simulink model "VehicleTest"  (Simulink 4.00)
settings: Solver=FixedStepDiscrete  StartTime=0.0  StopTime=GlobalStopTime  FixedStep=GlobalSampleTime  RelTol=1e-3
undefined symbols (not defined in the file): EntityTypes, g_EnableTarget, g_VehicleInputFiles, GlobalSampleTime, GSensorRollLimitDeg, OptionSaveDataAVDS, OptionSaveDataPlot, TargetStates, WaypointDefinitions
settings Model: Creator=mitchejw  LastModifiedBy=rasmussj  SaveTime=off  SaveOutput=off  ExtModeAutoUpdateStatusClock=off

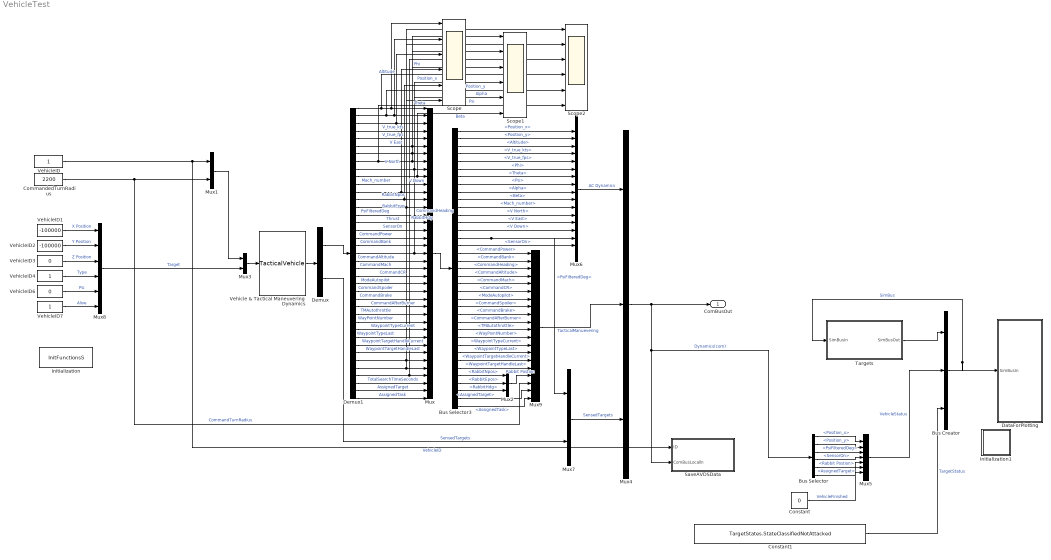
== system VehicleTest ==
  Bus Creator : BusCreator  Inputs=3
  Bus Selector : BusSelector  OutputSignals=AC Dynamics.Position_x,AC Dynamics.Position_y,AC Dynamics.PsiFilteredDeg,AC Dynamics.SensorOn,TacticalManuevering.Rabbit Postion,TacticalManuevering.AssignedTarget  MuxedOutput=off
  Bus Selector3 : BusSelector  OutputSignals=Position_x,Position_y,Altitude,V_true_kts,V_true_fps,Phi,Theta,Psi,Alpha,Beta,Mach_number,V North,V East,V Down,PsiFilteredDeg,SensorOn,CommandPower,CommandBank,CommandHeading,CommandAltitude,CommandMach,CommandCR,ModeAutopilot,CommandSpoiler,CommandBrake,CommandAfterBurner,TMAutothrottle,WayPointNumber,WaypointTypeCurrent,WaypointTypeLast,WaypointTargetHandleCurrent,WaypointTargetHandleLast,RabbitNpos,RabbitEpos,RabbitHdg,AssignedTarget,AssignedTask  MuxedOutput=off
  CommandedTurnRadius : Constant  Value=2200
  Constant : Constant  Value=0
  Constant1 : Constant  Value=TargetStates.StateClassifiedNotAttacked
  DataForPlotting : Subsystem  Priority=5
      settings: RTWFcnNameOpts=Auto  RTWFileNameOpts=Auto
  Demux : Demux  Outputs=[39 1]  BusSelectionMode=off
  Demux1 : Demux  Outputs=39  BusSelectionMode=off
  Initialization : S-Function  FunctionName=InitFunctionsS  PortCounts=[]  SFunctionModules=''
  Initialization1 : Subsystem  Priority=1
      settings: RTWFcnNameOpts=Auto  RTWFileNameOpts=Auto
  Mux : Mux  Inputs="[1 1 1 1 1 1 1 1 1 1 1 1 1 1 1 1 1 1 1 1  1 1 1 1 1 1 1 1 1 1  1 1 1 1 1 1 1 1 1]"
  Mux1 : Mux  Inputs=2
  Mux2 : Mux  Inputs=3
  Mux3 : Mux  Inputs=2
  Mux4 : Mux  Inputs=3
  Mux5 : Mux  Inputs=7
  Mux6 : Mux  Inputs=16
  Mux7 : Mux  Inputs=2
  Mux8 : Mux  Inputs=6
  Mux9 : Mux  Inputs=[1 1 1 1 1 1 1 1 1 1 1 1 1 1 1 1 3 1 1 1]
  SaveAVDSData : Subsystem
      settings: RTWFcnNameOpts=Auto  RTWFileNameOpts=Auto
  Scope : Scope  NumInputPorts=6
      settings: TimeRange=auto  YMin=0~-150~-1000~0~-125~-175  YMax=2000~50~0~400~100~100  SaveToWorkspace=off  SaveName=ScopeData  LimitDataPoints=on  MaxDataPoints=5000
  Scope1 : Scope  NumInputPorts=6
      settings: TimeRange=auto  YMin=-10~-1~-1~-0.8~-0.4~0  YMax=70~0.5~0.75~0.4~0.4~400  SaveToWorkspace=off  LimitDataPoints=on  MaxDataPoints=5000
  Scope2 : Scope  NumInputPorts=6
      settings: TimeRange=auto  YMin=-2500~-8000~-1.75~0~-6000~0  YMax=25000~0~0~27500~500~200  SaveToWorkspace=off  SaveName=ScopeData2  LimitDataPoints=on  MaxDataPoints=5000
  Targets : Subsystem  Priority=2  TreatAsAtomicUnit=on
      settings: RTWFcnNameOpts=Auto  RTWFileNameOpts=Auto
  Vehicle & Tactical Maneuvering  Dynamics : S-Function  FunctionName=TacticalVehicle  Parameters=0,1,GSensorRollLimitDeg,WaypointDefinitions.NumberEntries,g_VehicleInputFiles  PortCounts=[]  SFunctionModules=''
  VehicleID : Constant  Value=1
  VehicleID1 : Constant  Value=-100000
  VehicleID2 : Constant  Value=-100000
  VehicleID3 : Constant  Value=0
  VehicleID4 : Constant  Value=1
  VehicleID6 : Constant  Value=0
  VehicleID7 : Constant  Value=1
  ComBusOut : Outport  Port=1
  wires:
  Mux3/1 -> Vehicle & Tactical Maneuvering  Dynamics/1
  Mux8/1 -> Mux3/2  "Target"
  Mux1/1 -> Mux3/1
  Vehicle & Tactical Maneuvering  Dynamics/1 -> Demux/1
  VehicleID/1 -> Mux1/1, SaveAVDSData/1(ID)  "VehicleID"
  CommandedTurnRadius/1 -> Mux1/2, Mux9/18  "CommandTurnRadius"
  Mux4/1 -> ComBusOut/1, SaveAVDSData/2(ComBusLocalln), Bus Selector/1  "Dynamics(com)"
  Mux7/1 -> Mux4/3  "SensedTargets"
  Demux/1 -> Demux1/1
  Demux/2 -> Mux7/2  "SensedTargets"
  Demux1/3 -> Mux/3, Scope/3  "Altitude"
  Demux1/1 -> Mux/1, Scope/1, Scope2/4  "Position_x"
  Demux1/2 -> Mux/2, Scope/2, Scope2/5  "Position_y"
  Demux1/4 -> Mux/4  "V_true_kts"
  Demux1/5 -> Mux/5  "V_true_fps"
  Demux1/6 -> Mux/6, Scope1/1  "Phi"
  Demux1/7 -> Mux/7, Scope1/2  "Theta"
  Demux1/8 -> Mux/8, Scope1/3, Scope2/6  "Psi"
  Demux1/9 -> Mux/9, Scope1/5  "Alpha"
  Demux1/10 -> Mux/10, Scope1/6  "Beta"
  Demux1/11 -> Mux/11  "Mach_number"
  Demux1/12 -> Mux/12, Scope/4  "V North"
  Demux1/13 -> Mux/13, Scope/5  "V East"
  Demux1/14 -> Mux/14, Scope/6  "V Down"
  Demux1/15 -> Mux/15  "PsiFilteredDeg"
  Demux1/16 -> Mux/16  "Thrust"
  Demux1/17 -> Mux/17  "SensorOn"
  Demux1/18 -> Mux/18  "CommandPower"
  Demux1/19 -> Mux/19  "CommandBank"
  Demux1/20 -> Mux/20, Scope1/4  "CommandHeading"
  Demux1/21 -> Mux/21  "CommandAltitude"
  Demux1/22 -> Mux/22  "CommandMach"
  Demux1/23 -> Mux/23  "CommandCR"
  Demux1/24 -> Mux/24  "ModeAutopilot"
  Demux1/25 -> Mux/25  "CommandSpoiler"
  Demux1/26 -> Mux/26  "CommandBrake"
  Demux1/27 -> Mux/27  "CommandAfterBurner"
  Demux1/28 -> Mux/28  "TMAutothrottle"
  Demux1/29 -> Mux/29  "WayPointNumber"
  Bus Selector3/1 -> Mux6/1  "<Position_x>"
  Bus Selector3/2 -> Mux6/2  "<Position_y>"
  Bus Selector3/3 -> Mux6/3  "<Altitude>"
  Bus Selector3/4 -> Mux6/4  "<V_true_kts>"
  Bus Selector3/5 -> Mux6/5  "<V_true_fps>"
  Bus Selector3/6 -> Mux6/6  "<Phi>"
  Bus Selector3/7 -> Mux6/7  "<Theta>"
  Bus Selector3/8 -> Mux6/8  "<Psi>"
  Bus Selector3/9 -> Mux6/9  "<Alpha>"
  Bus Selector3/10 -> Mux6/10  "<Beta>"
  Bus Selector3/11 -> Mux6/11  "<Mach_number>"
  Bus Selector3/12 -> Mux6/12  "<V North>"
  Bus Selector3/13 -> Mux6/13  "<V East>"
  Bus Selector3/14 -> Mux6/14  "<V Down>"
  Bus Selector3/15 -> Mux6/15, Mux7/1  "<PsiFilteredDeg>"
  Mux6/1 -> Mux4/1  "AC Dynamics"
  Bus Selector3/16 -> Mux6/16  "<SensorOn>"
  Mux/1 -> Bus Selector3/1
  Bus Selector3/17 -> Mux9/1  "<CommandPower>"
  Bus Selector3/18 -> Mux9/2  "<CommandBank>"
  Bus Selector3/19 -> Mux9/3  "<CommandHeading>"
  Bus Selector3/20 -> Mux9/4  "<CommandAltitude>"
  Bus Selector3/21 -> Mux9/5  "<CommandMach>"
  Bus Selector3/22 -> Mux9/6  "<CommandCR>"
  Bus Selector3/23 -> Mux9/7  "<ModeAutopilot>"
  Bus Selector3/24 -> Mux9/8  "<CommandSpoiler>"
  Bus Selector3/25 -> Mux9/9  "<CommandBrake>"
  Bus Selector3/26 -> Mux9/10  "<CommandAfterBurner>"
  Bus Selector3/27 -> Mux9/11  "<TMAutothrottle>"
  Bus Selector3/28 -> Mux9/12  "<WayPointNumber>"
  Mux9/1 -> Mux4/2  "TacticalManuevering"
  Demux1/34 -> Mux/34, Scope2/1  "RabbitNpos"
  Demux1/30 -> Mux/30  "WaypointTypeCurrent"
  Demux1/31 -> Mux/31  "WaypointTypeLast"
  Demux1/32 -> Mux/32  "WaypointTargetHandleCurrent"
  Demux1/33 -> Mux/33  "WaypointTargetHandleLast"
  Bus Selector3/29 -> Mux9/13  "<WaypointTypeCurrent>"
  Bus Selector3/30 -> Mux9/14  "<WaypointTypeLast>"
  Demux1/35 -> Mux/35, Scope2/2  "RabbitEpos"
  Demux1/36 -> Mux/36, Scope2/3  "RabbitHdg"
  Mux2/1 -> Mux9/17  "Rabbit Postion"
  Bus Selector3/35 -> Mux2/3  "<RabbitHdg>"
  Bus Selector3/34 -> Mux2/2  "<RabbitEpos>"
  Bus Selector3/33 -> Mux2/1  "<RabbitNpos>"
  Bus Selector3/32 -> Mux9/16  "<WaypointTargetHandleLast>"
  Bus Selector3/31 -> Mux9/15  "<WaypointTargetHandleCurrent>"
  Demux1/37 -> Mux/37  "TotalSearchTimeSeconds"
  Demux1/38 -> Mux/38  "AssignedTarget"
  Demux1/39 -> Mux/39  "AssignedTask"
  Bus Selector3/37 -> Mux9/20  "<AssignedTask>"
  Bus Selector3/36 -> Mux9/19  "<AssignedTarget>"
  VehicleID1/1 -> Mux8/1  "X Position"
  VehicleID2/1 -> Mux8/2  "Y Position"
  VehicleID3/1 -> Mux8/3  "Z Position"
  VehicleID6/1 -> Mux8/5  "Psi"
  VehicleID4/1 -> Mux8/4  "Type"
  VehicleID7/1 -> Mux8/6  "Alive"
  Targets/1(SimBusOut) -> Bus Creator/1
  Bus Creator/1 -> Targets/1(SimBusIn), DataForPlotting/1(SimBusIn)  "SimBus"
  Bus Selector/1 -> Mux5/1  "<Position_x>"
  Bus Selector/2 -> Mux5/2  "<Position_y>"
  Bus Selector/3 -> Mux5/3  "<PsiFilteredDeg>"
  Bus Selector/4 -> Mux5/4  "<SensorOn>"
  Bus Selector/5 -> Mux5/5  "<Rabbit Postion>"
  Bus Selector/6 -> Mux5/6  "<AssignedTarget>"
  Mux5/1 -> Bus Creator/2  "VehicleStatus"
  Constant/1 -> Mux5/7  "VehicleFinished"
  Constant1/1 -> Bus Creator/3  "TargetStatus"

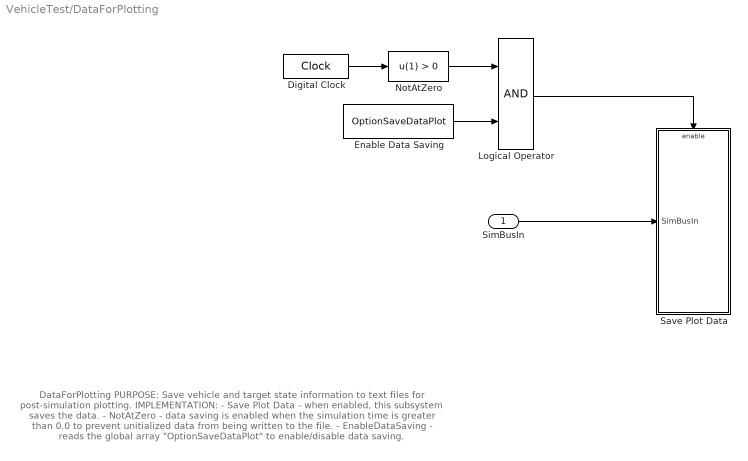
== system VehicleTest/DataForPlotting ==
  note: DataForPlotting
      |
      | PURPOSE: Save vehicle and target state information to text files for
      |      post-simulation plotting.
      |
      | IMPLEMENTATION:
      | - Save Plot Data - when enabled, this subsystem saves the data.
      | - NotAtZero - data saving is enabled when the simulation time is greater
      |      than 0.0 to prevent unitialized data from being written to the file.
      | - EnableDataSaving - reads the global array "OptionSaveDataPlot" to
      |      enable/disable data saving.
  SimBusIn : Inport  Port=1  LatchInput=off  SampleTime=GlobalSampleTime
  Digital Clock : DigitalClock  SampleTime=GlobalSampleTime
  Enable Data Saving : Constant  Value=OptionSaveDataPlot
  Logical Operator : Logic  Operator=AND  Inputs=2
  NotAtZero : Fcn  Expr=u(1) > 0
  Save Plot Data : Subsystem  TreatAsAtomicUnit=on
      settings: RTWFcnNameOpts=Auto  RTWFileNameOpts=Auto
  wires:
  Digital Clock/1 -> NotAtZero/1
  SimBusIn/1 -> Save Plot Data/1(SimBusIn)
  NotAtZero/1 -> Logical Operator/1
  Enable Data Saving/1 -> Logical Operator/2
  Logical Operator/1 -> Save Plot Data/Enable

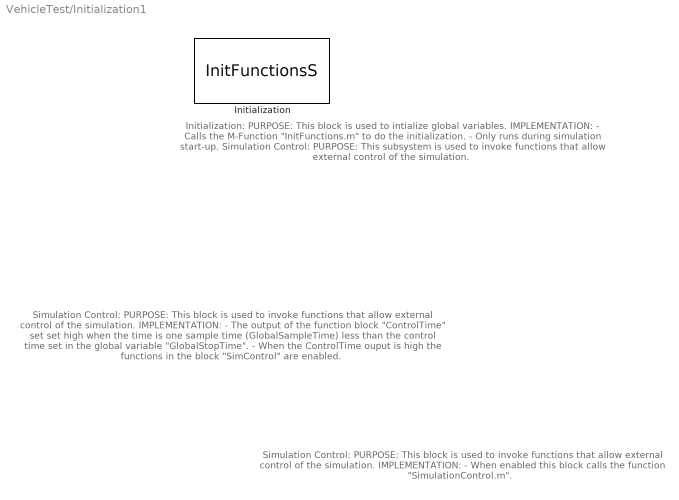
== system VehicleTest/Initialization1 ==
  note: Initialization:
      | PURPOSE: This block is used to intialize global variables.
      | IMPLEMENTATION:
      | - Calls the M-Function "InitFunctions.m" to do the initialization.
      | - Only runs during simulation start-up.
      |
      | Simulation Control:
      | PURPOSE: This subsystem is used to invoke functions that
      | allow external control of the simulation.
  note: Simulation Control:
      |
      | PURPOSE: This block is used to invoke functions that
      | allow external control of the simulation.
      | IMPLEMENTATION:
      | - The output of the function block  "ControlTime" set set high when
      | the time is one sample time (GlobalSampleTime) less than the control
      | time set in the global variable "GlobalStopTime".
      | - When the ControlTime ouput is high the functions in the
      | block "SimControl" are enabled.
  note: Simulation Control:
      |
      | PURPOSE: This block is used to invoke functions that
      | allow external control of the simulation.
      | IMPLEMENTATION:
      | - When enabled this block calls the function "SimulationControl.m".
  Initialization : S-Function  FunctionName=InitFunctionsS  PortCounts=[]  SFunctionModules=''

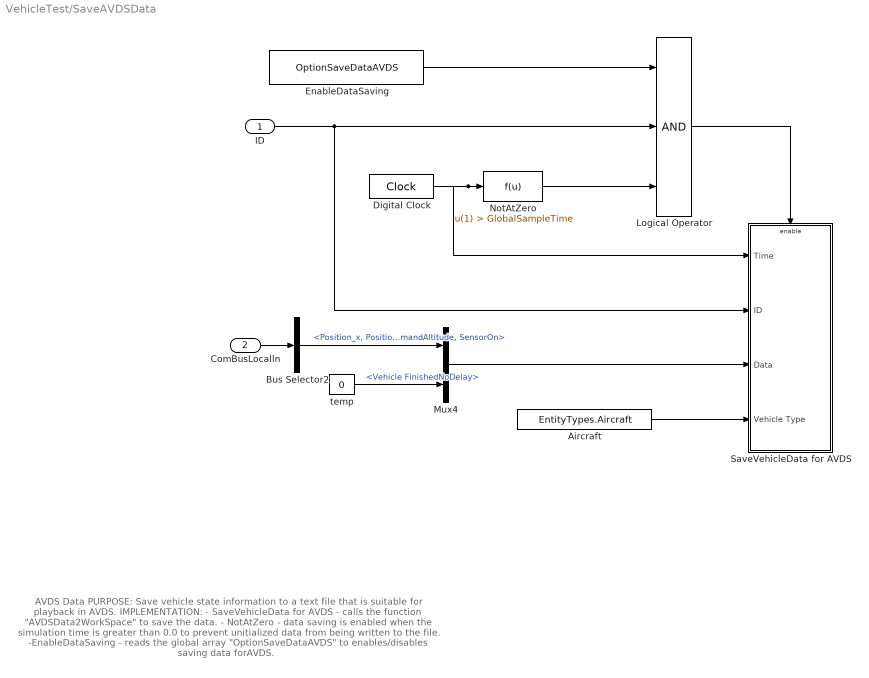
== system VehicleTest/SaveAVDSData ==
  note: AVDS Data
      |
      | PURPOSE: Save vehicle state information to a
      | text file that is suitable for playback in AVDS.
      |
      | IMPLEMENTATION:
      | - SaveVehicleData for AVDS - calls the function "AVDSData2WorkSpace"
      |      to save the data.
      | - NotAtZero - data saving is enabled when the simulation time is greater
      |      than 0.0 to prevent unitialized data from being written to the file.
      | -EnableDataSaving - reads the global array "OptionSaveDataAVDS" to
      |      enables/disables saving data forAVDS.
  ID : Inport  Port=1  LatchInput=off  SampleTime=GlobalSampleTime
  ComBusLocalln : Inport  Port=2  LatchInput=off  SampleTime=GlobalSampleTime
  Aircraft : Constant  Value=EntityTypes.Aircraft
  Bus Selector2 : BusSelector  OutputSignals=AC Dynamics.Position_x,AC Dynamics.Position_y,AC Dynamics.Altitude,AC Dynamics.Phi,AC Dynamics.Theta,AC Dynamics.Psi,AC Dynamics.Alpha,AC Dynamics.Beta,AC Dynamics.V_true_fps,AC Dynamics.Mach_number,TacticalManuevering.AssignedTarget,TacticalManuevering.AssignedTask,TacticalManuevering.Rabbit Postion,TacticalManuevering.CommandAltitude,AC Dynamics.SensorOn  MuxedOutput=on
  Digital Clock : DigitalClock  SampleTime=GlobalSampleTime
  "EnableDataSaving " : Constant  Value=OptionSaveDataAVDS
  Logical Operator : Logic  Operator=AND  Inputs=3
  Mux4 : Mux  Inputs=2
  NotAtZero : Fcn  Expr=u(1) > GlobalSampleTime
  SaveVehicleData for AVDS : Subsystem  TreatAsAtomicUnit=on
      settings: RTWFcnNameOpts=Auto  RTWFileNameOpts=Auto
  temp : Constant  Value=0
  wires:
  Mux4/1 -> SaveVehicleData for AVDS/3(Data)
  temp/1 -> Mux4/2  "<Vehicle FinishedNoDelay>"
  Bus Selector2/1 -> Mux4/1  "<Position_x, Position_y, Altitude, Phi, Theta, Psi, Alpha, Beta, V_true_fps, Mach_number, AssignedTarget, AssignedTask, Rabbit Postion, CommandAltitude, SensorOn>"
  "EnableDataSaving "/1 -> Logical Operator/1
  Logical Operator/1 -> SaveVehicleData for AVDS/Enable
  ID/1 -> Logical Operator/2, SaveVehicleData for AVDS/2(ID)
  ComBusLocalln/1 -> Bus Selector2/1
  Digital Clock/1 -> NotAtZero/1, SaveVehicleData for AVDS/1(Time)
  Aircraft/1 -> SaveVehicleData for AVDS/4(Vehicle Type)
  NotAtZero/1 -> Logical Operator/3

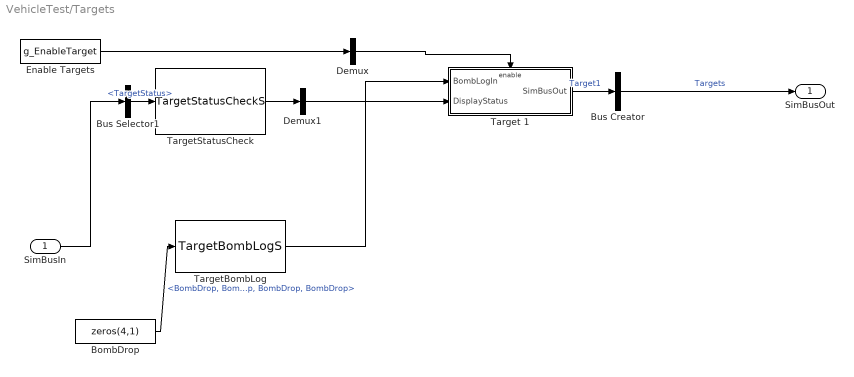
== system VehicleTest/Targets ==
  SimBusIn : Inport  Port=1  LatchInput=off  SampleTime=GlobalSampleTime
  BombDrop : Constant  Value=zeros(4,1)
  Bus Creator : BusCreator  Inputs=1
  Bus Selector1 : BusSelector  OutputSignals=TargetStatus  MuxedOutput=on
  Demux : Demux  Outputs=1  BusSelectionMode=off
  Demux1 : Demux  Outputs=1  BusSelectionMode=off
  Enable Targets : Constant  Value=g_EnableTarget
  Target 1 : Subsystem  AncestorBlock=cooperative/Target 1  TreatAsAtomicUnit=on
      settings: RTWFcnNameOpts=Auto  RTWFileNameOpts=Auto
  TargetBombLog : S-Function  FunctionName=TargetBombLogS  PortCounts=[]  SFunctionModules=''
  TargetStatusCheck : S-Function  FunctionName=TargetStatusCheckS  PortCounts=[]  SFunctionModules=''
  SimBusOut : Outport  Port=1
  wires:
  SimBusIn/1 -> Bus Selector1/1
  Bus Creator/1 -> SimBusOut/1  "Targets"
  Target 1/1(SimBusOut) -> Bus Creator/1  "Target1"
  Enable Targets/1 -> Demux/1
  BombDrop/1 -> TargetBombLog/1  "<BombDrop, BombDrop, BombDrop, BombDrop, BombDrop, BombDrop, BombDrop, BombDrop>"
  TargetBombLog/1 -> Target 1/1(BombLogIn)
  Bus Selector1/1 -> TargetStatusCheck/1  "<TargetStatus>"
  TargetStatusCheck/1 -> Demux1/1
  Demux1/1 -> Target 1/2(DisplayStatus)
  Demux/1 -> Target 1/Enable

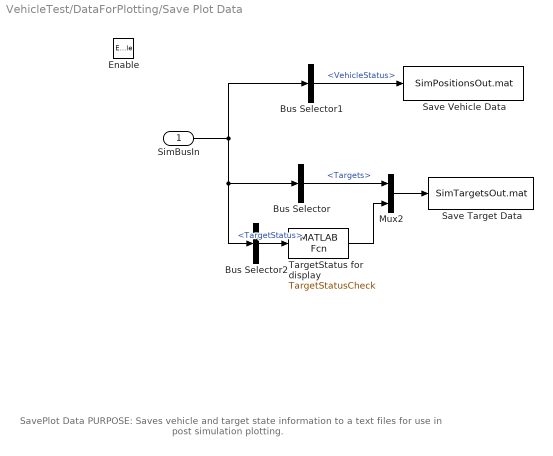
== system VehicleTest/DataForPlotting/Save Plot Data ==
  note: SavePlot Data
      |
      | PURPOSE: Saves vehicle and target state information to a text files for use
      |      in post simulation plotting.
  SimBusIn : Inport  Port=1  LatchInput=off  SampleTime=GlobalSampleTime
  Enable : EnablePort
  Bus Selector : BusSelector  OutputSignals=Targets  MuxedOutput=on
  Bus Selector1 : BusSelector  OutputSignals=VehicleStatus  MuxedOutput=on
  Bus Selector2 : BusSelector  OutputSignals=TargetStatus  MuxedOutput=on
  Mux2 : Mux  Inputs=2
  Save Target Data : ToFile  Filename=SimTargetsOut.mat  MatrixName=TargetPositions  SampleTime=GlobalSampleTime
  Save Vehicle Data : ToFile  Filename=SimPositionsOut.mat  MatrixName=XYPositions  SampleTime=GlobalSampleTime
  TargetStatus for display : MATLABFcn  MATLABFcn=TargetStatusCheck  OutputDimensions=-1  OutputSignalType=auto  Output1D=on
  wires:
  Bus Selector1/1 -> Save Vehicle Data/1  "<VehicleStatus>"
  SimBusIn/1 -> Bus Selector/1, Bus Selector2/1, Bus Selector1/1
  TargetStatus for display/1 -> Mux2/2
  Bus Selector2/1 -> TargetStatus for display/1  "<TargetStatus>"
  Bus Selector/1 -> Mux2/1  "<Targets>"
  Mux2/1 -> Save Target Data/1

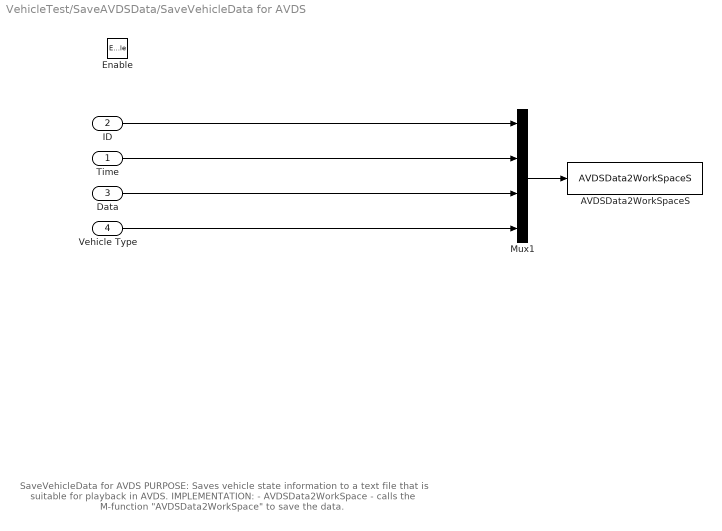
== system VehicleTest/SaveAVDSData/SaveVehicleData for AVDS ==
  note: SaveVehicleData for AVDS
      |
      | PURPOSE: Saves vehicle state information to a text file that is suitable
      |      for playback in AVDS.
      | IMPLEMENTATION:
      | - AVDSData2WorkSpace - calls the M-function "AVDSData2WorkSpace"
      |      to save the data.
  Time : Inport  Port=1  LatchInput=off  SampleTime=GlobalSampleTime
  ID : Inport  Port=2  LatchInput=off  SampleTime=GlobalSampleTime
  Data : Inport  Port=3  LatchInput=off  SampleTime=GlobalSampleTime
  Vehicle Type : Inport  Port=4  LatchInput=off  SampleTime=GlobalSampleTime
  Enable : EnablePort
  AVDSData2WorkSpaceS : S-Function  FunctionName=AVDSData2WorkSpaceS  PortCounts=[]  SFunctionModules=''
  Mux1 : Mux  Inputs=4
  wires:
  Mux1/1 -> AVDSData2WorkSpaceS/1
  Time/1 -> Mux1/2
  ID/1 -> Mux1/1
  Data/1 -> Mux1/3
  Vehicle Type/1 -> Mux1/4

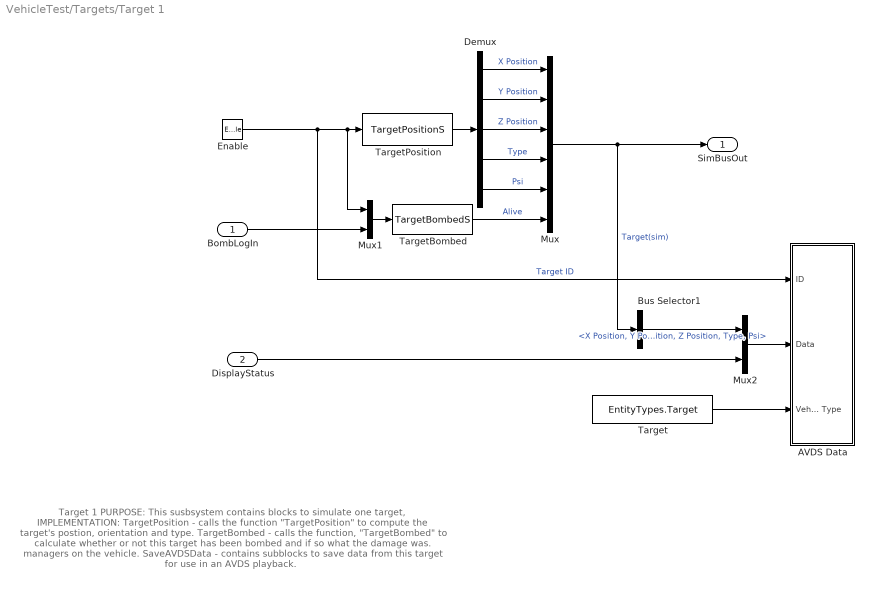
== system VehicleTest/Targets/Target 1 ==
  note: Target 1
      |
      | PURPOSE: This susbsystem contains blocks to simulate one target,
      |
      | IMPLEMENTATION:
      | TargetPosition - calls the function "TargetPosition" to compute the target's postion,
      |      orientation and type.
      | TargetBombed - calls the function, "TargetBombed" to calculate whether or not this
      |      target has been bombed and if so what the damage was.
      |      managers on the vehicle.
      | SaveAVDSData - contains subblocks to save data from this target for use
      |     in an AVDS playback.
  BombLogIn : Inport  Port=1  LatchInput=off  SampleTime=GlobalSampleTime
  DisplayStatus : Inport  Port=2  LatchInput=off  SampleTime=GlobalSampleTime
  Enable : EnablePort  StatesWhenEnabling=reset  ShowOutputPort=on
  AVDS Data : Subsystem
      settings: RTWFcnNameOpts=Auto  RTWFileNameOpts=Auto
  Bus Selector1 : BusSelector  OutputSignals=X Position,Y Position,Z Position,Type,Psi  MuxedOutput=on
  Demux : Demux  Outputs=5  BusSelectionMode=off
  Mux : Mux  Inputs=6
  Mux1 : Mux  Inputs=2
  Mux2 : Mux  Inputs=2
  Target : Constant  Value=EntityTypes.Target
  TargetBombed : S-Function  FunctionName=TargetBombedS  PortCounts=[]  SFunctionModules=''
  TargetPosition : S-Function  FunctionName=TargetPositionS  PortCounts=[]  SFunctionModules=''
  SimBusOut : Outport  Port=1  InitialOutput=[1e7 1e7 0 1 -1 -1]
  wires:
  Enable/1 -> AVDS Data/1(ID), Mux1/1, TargetPosition/1  "Target ID"
  TargetPosition/1 -> Demux/1
  Target/1 -> AVDS Data/3(Vehicle Type)
  Bus Selector1/1 -> Mux2/1  "<X Position, Y Position, Z Position, Type, Psi>"
  Demux/1 -> Mux/1  "X Position"
  Demux/2 -> Mux/2  "Y Position"
  Demux/3 -> Mux/3  "Z Position"
  Mux/1 -> SimBusOut/1, Bus Selector1/1  "Target(sim)"
  Demux/5 -> Mux/5  "Psi"
  BombLogIn/1 -> Mux1/2
  Demux/4 -> Mux/4  "Type"
  TargetBombed/1 -> Mux/6  "Alive"
  Mux1/1 -> TargetBombed/1
  Mux2/1 -> AVDS Data/2(Data)
  DisplayStatus/1 -> Mux2/2

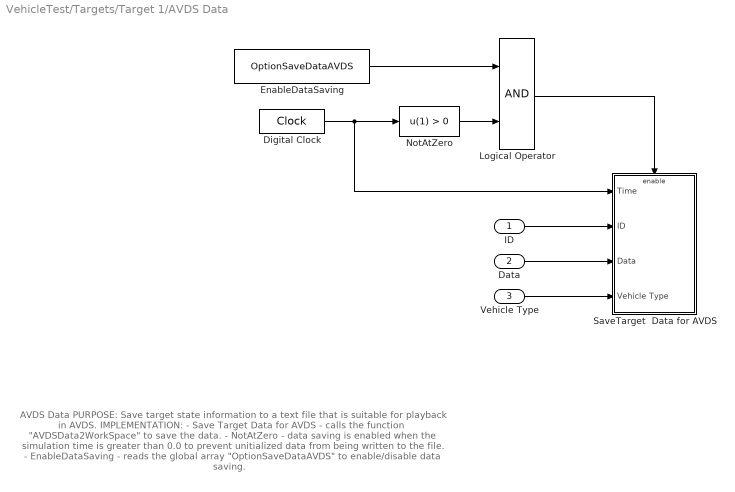
== system VehicleTest/Targets/Target 1/AVDS Data ==
  note: AVDS Data
      |
      | PURPOSE: Save target state information to a text file that is suitable
      |      for playback in AVDS.
      |
      | IMPLEMENTATION:
      | - Save Target Data for AVDS - calls the function "AVDSData2WorkSpace"
      |      to save the data.
      | - NotAtZero - data saving is enabled when the simulation time is greater
      |      than 0.0 to prevent unitialized data from being written to the file.
      | - EnableDataSaving - reads the global array "OptionSaveDataAVDS" to
      |      enable/disable data saving.
  ID : Inport  Port=1  LatchInput=off  SampleTime=GlobalSampleTime
  Data : Inport  Port=2  LatchInput=off  SampleTime=GlobalSampleTime
  Vehicle Type : Inport  Port=3  LatchInput=off  SampleTime=GlobalSampleTime
  Digital Clock : DigitalClock  SampleTime=GlobalSampleTime
  EnableDataSaving : Constant  Value=OptionSaveDataAVDS
  Logical Operator : Logic  Operator=AND  Inputs=2
  NotAtZero : Fcn  Expr=u(1) > 0
  SaveTarget  Data for AVDS : Subsystem  TreatAsAtomicUnit=on
      settings: RTWFcnNameOpts=Auto  RTWFileNameOpts=Auto
  wires:
  ID/1 -> SaveTarget  Data for AVDS/2(ID)
  Data/1 -> SaveTarget  Data for AVDS/3(Data)
  Digital Clock/1 -> NotAtZero/1, SaveTarget  Data for AVDS/1(Time)
  Vehicle Type/1 -> SaveTarget  Data for AVDS/4(Vehicle Type)
  NotAtZero/1 -> Logical Operator/2
  Logical Operator/1 -> SaveTarget  Data for AVDS/Enable
  EnableDataSaving/1 -> Logical Operator/1

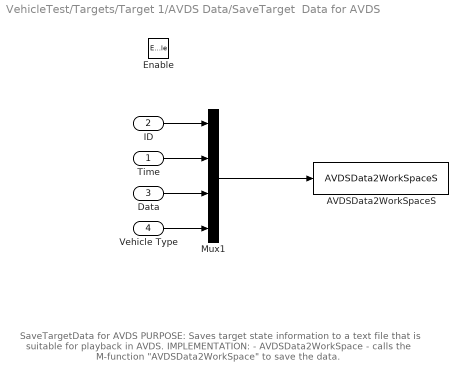
== system VehicleTest/Targets/Target 1/AVDS Data/SaveTarget  Data for AVDS ==
  note: SaveTargetData for AVDS
      |
      | PURPOSE: Saves target state information to a text file that is suitable
      |      for playback in AVDS.
      | IMPLEMENTATION:
      | - AVDSData2WorkSpace - calls the M-function "AVDSData2WorkSpace"
      |      to save the data.
  Time : Inport  Port=1  LatchInput=off  SampleTime=GlobalSampleTime
  ID : Inport  Port=2  LatchInput=off  SampleTime=GlobalSampleTime
  Data : Inport  Port=3  LatchInput=off  SampleTime=GlobalSampleTime
  Vehicle Type : Inport  Port=4  LatchInput=off  SampleTime=GlobalSampleTime
  Enable : EnablePort
  AVDSData2WorkSpaceS : S-Function  FunctionName=AVDSData2WorkSpaceS  PortCounts=[]  SFunctionModules=''
  Mux1 : Mux  Inputs=4
  wires:
  Mux1/1 -> AVDSData2WorkSpaceS/1
  Time/1 -> Mux1/2
  ID/1 -> Mux1/1
  Data/1 -> Mux1/3
  Vehicle Type/1 -> Mux1/4
